simulink model "Simulation"  (R2023b)
settings: Solver=VariableStepAuto  StartTime=0.0  StopTime=1  RelTol=1e-3
values from neighbouring files (symbols this model uses):
  Adj = Adj1'    [graph_plot.m]
  G = digraph(Adj)    [graph_plot.m]
undefined symbols (not defined in the file or in its folder): A, B, c, C, F, K, Ko, L1, x0_0, xi_0
libraries: simulink x7
settings Model: Creator=fedpa  LastModifiedBy=fedpa

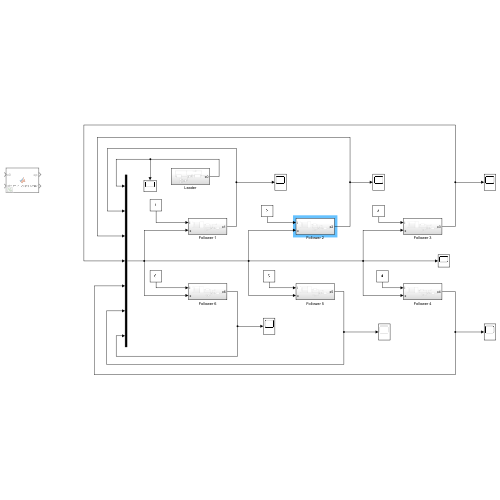
[thumbnail: Simulink's stored preview of the top-level diagram]
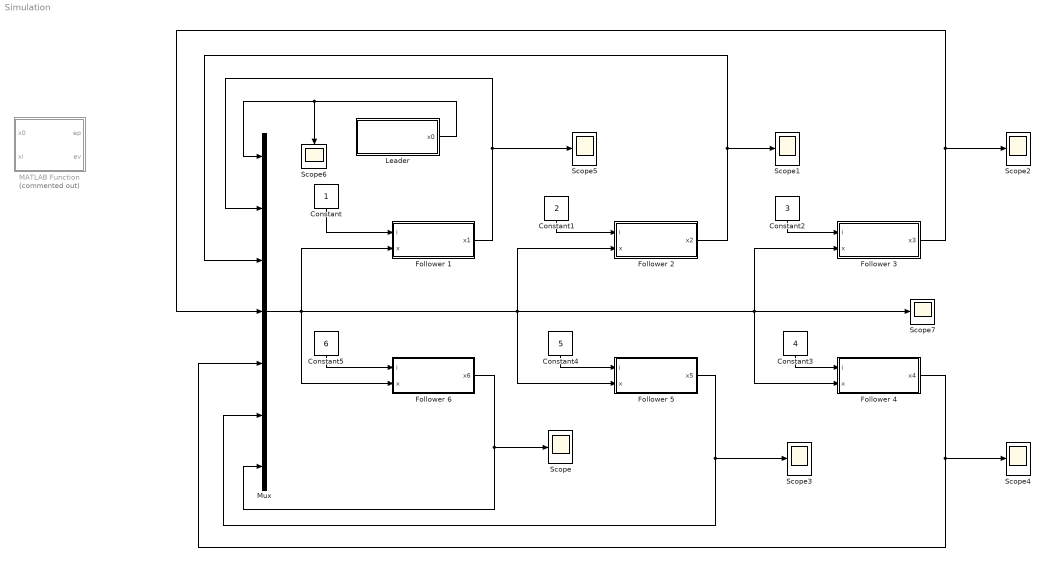
== system Simulation ==
  Constant : Constant
  Constant1 : Constant  Value=2
  Constant2 : Constant  Value=3
  Constant3 : Constant  Value=4
  Constant4 : Constant  Value=5
  Constant5 : Constant  Value=6
  Follower 1 : Subsystem
  Follower 2 : Subsystem
  Follower 3 : Subsystem
  Follower 4 : Subsystem
  Follower 5 : Subsystem
  Follower 6 : Subsystem
  Leader : Subsystem
  MATLAB Function : MATLAB Function  Commented=on  TreatAsAtomicUnit=on
  Mux : Mux  Inputs=7
  Scope{,1..7} (8 alike) : Scope
  wires:
  Constant3/1 -> Follower 4/1(i)
  Follower 3/1(x3) -> Scope2/1, Mux/4
  Follower 4/1(x4) -> Mux/5, Scope4/1
  Constant4/1 -> Follower 5/1(i)
  Constant5/1 -> Follower 6/1(i)
  Mux/1 -> Follower 1/2(x), Follower 5/2(x), Follower 2/2(x), Follower 4/2(x), Follower 3/2(x), Scope7/1, Follower 6/2(x)
  Follower 5/1(x5) -> Scope3/1, Mux/6
  Constant2/1 -> Follower 3/1(i)
  Follower 1/1(x1) -> Mux/2, Scope5/1
  Follower 2/1(x2) -> Mux/3, Scope1/1
  Constant/1 -> Follower 1/1(i)
  Constant1/1 -> Follower 2/1(i)
  Leader/1(x0) -> Mux/1, Scope6/1
  Follower 6/1(x6) -> Mux/7, Scope/1

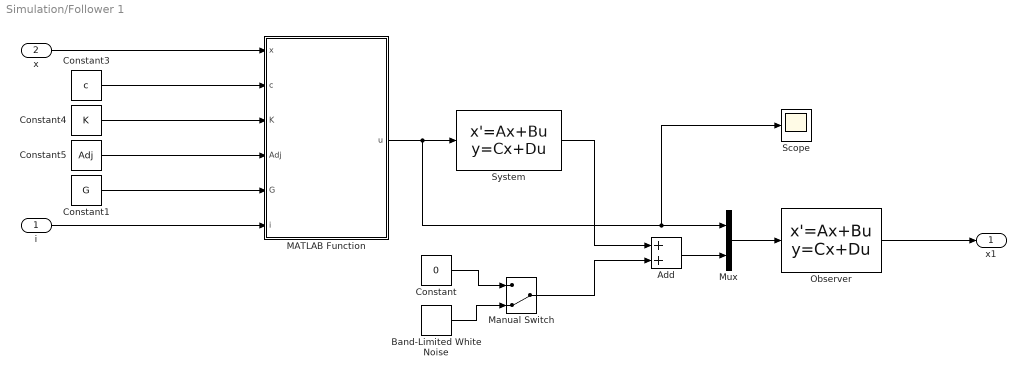
== system Simulation/Follower 1 ==
  i : Inport
  x : Inport  Port=2
  Add : Sum
  Band-Limited White Noise : simulink/Sources/Band-Limited White Noise  Cov=dis  Ts=0.1  seed=[23341]
  Constant : Constant  Value=0
  Constant1 : Constant  Value=G  VectorParams1D=off
  Constant3 : Constant  Value=c
  Constant4 : Constant  Value=K  VectorParams1D=off
  Constant5 : Constant  Value=Adj  VectorParams1D=off
  MATLAB Function : MATLAB Function  TreatAsAtomicUnit=on
  Manual Switch : ManualSwitch  CurrentSetting=0
  Mux : Mux  Inputs=2
  Observer : StateSpace  A=A-B*Ko-c*F*C  B=[B c*F]  C=eye(2)  D=zeros(2,2)  InitialCondition=0
  Scope : Scope
  System : StateSpace  A=A-B*Ko  B=B  C=C  D=0  InitialCondition=xi_0
  x1 : Outport
  wires:
  MATLAB Function/1(u) -> System/1, Scope/1, Mux/1
  Mux/1 -> Observer/1
  Observer/1 -> x1/1
  Constant4/1 -> MATLAB Function/3(K)
  i/1 -> MATLAB Function/6(i)
  Constant3/1 -> MATLAB Function/2(c)
  Constant1/1 -> MATLAB Function/5(G)
  Constant5/1 -> MATLAB Function/4(Adj)
  x/1 -> MATLAB Function/1(x)
  Add/1 -> Mux/2
  System/1 -> Add/1
  Manual Switch/1 -> Add/2
  Constant/1 -> Manual Switch/1
  Band-Limited White Noise/1 -> Manual Switch/2

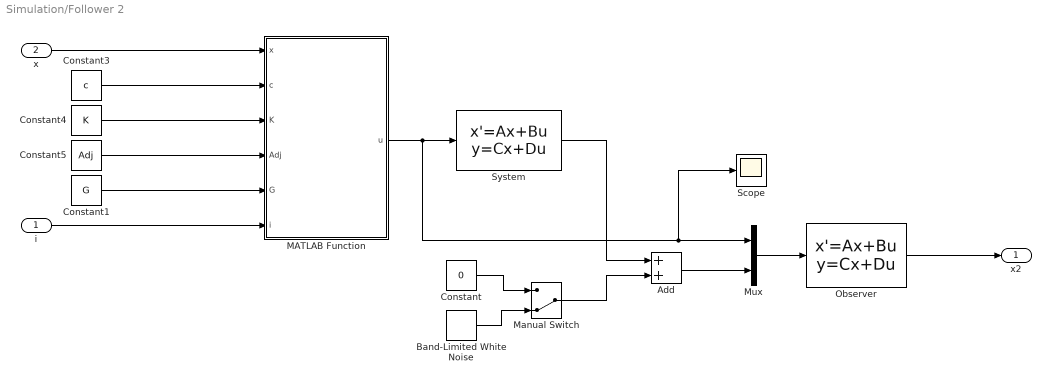
== system Simulation/Follower 2 ==
  i : Inport
  x : Inport  Port=2
  Add : Sum
  Band-Limited White Noise : simulink/Sources/Band-Limited White Noise  Cov=dis  Ts=0.1  seed=[23341]
  Constant : Constant  Value=0
  Constant1 : Constant  Value=G  VectorParams1D=off
  Constant3 : Constant  Value=c
  Constant4 : Constant  Value=K  VectorParams1D=off
  Constant5 : Constant  Value=Adj  VectorParams1D=off
  MATLAB Function : MATLAB Function  TreatAsAtomicUnit=on
  Manual Switch : ManualSwitch  CurrentSetting=0
  Mux : Mux  Inputs=2
  Observer : StateSpace  A=A-B*Ko-c*F*C  B=[B c*F]  C=eye(2)  D=zeros(2,2)  InitialCondition=0
  Scope : Scope
  System : StateSpace  A=A-B*Ko  B=B  C=C  D=0  InitialCondition=xi_0
  x2 : Outport
  wires:
  MATLAB Function/1(u) -> Scope/1, Mux/1, System/1
  Mux/1 -> Observer/1
  Observer/1 -> x2/1
  Constant4/1 -> MATLAB Function/3(K)
  i/1 -> MATLAB Function/6(i)
  Constant3/1 -> MATLAB Function/2(c)
  Constant1/1 -> MATLAB Function/5(G)
  Constant5/1 -> MATLAB Function/4(Adj)
  x/1 -> MATLAB Function/1(x)
  Add/1 -> Mux/2
  System/1 -> Add/1
  Manual Switch/1 -> Add/2
  Constant/1 -> Manual Switch/1
  Band-Limited White Noise/1 -> Manual Switch/2

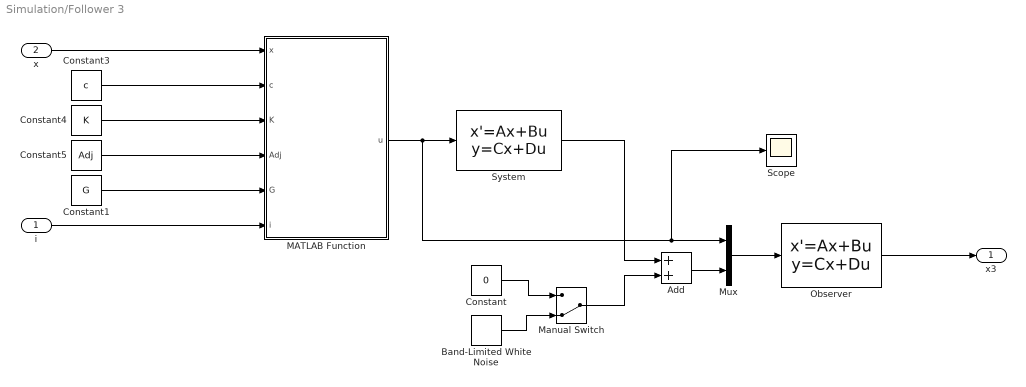
== system Simulation/Follower 3 ==
  i : Inport
  x : Inport  Port=2
  Add : Sum
  Band-Limited White Noise : simulink/Sources/Band-Limited White Noise  Cov=dis  Ts=0.1  seed=[23341]
  Constant : Constant  Value=0
  Constant1 : Constant  Value=G  VectorParams1D=off
  Constant3 : Constant  Value=c
  Constant4 : Constant  Value=K  VectorParams1D=off
  Constant5 : Constant  Value=Adj  VectorParams1D=off
  MATLAB Function : MATLAB Function  TreatAsAtomicUnit=on
  Manual Switch : ManualSwitch  CurrentSetting=0
  Mux : Mux  Inputs=2
  Observer : StateSpace  A=A-B*Ko-c*F*C  B=[B c*F]  C=eye(2)  D=zeros(2,2)  InitialCondition=0
  Scope : Scope
  System : StateSpace  A=A-B*Ko  B=B  C=C  D=0  InitialCondition=xi_0
  x3 : Outport
  wires:
  MATLAB Function/1(u) -> System/1, Scope/1, Mux/1
  Mux/1 -> Observer/1
  Observer/1 -> x3/1
  Constant4/1 -> MATLAB Function/3(K)
  i/1 -> MATLAB Function/6(i)
  Constant3/1 -> MATLAB Function/2(c)
  Constant1/1 -> MATLAB Function/5(G)
  Constant5/1 -> MATLAB Function/4(Adj)
  x/1 -> MATLAB Function/1(x)
  Add/1 -> Mux/2
  Manual Switch/1 -> Add/2
  System/1 -> Add/1
  Constant/1 -> Manual Switch/1
  Band-Limited White Noise/1 -> Manual Switch/2

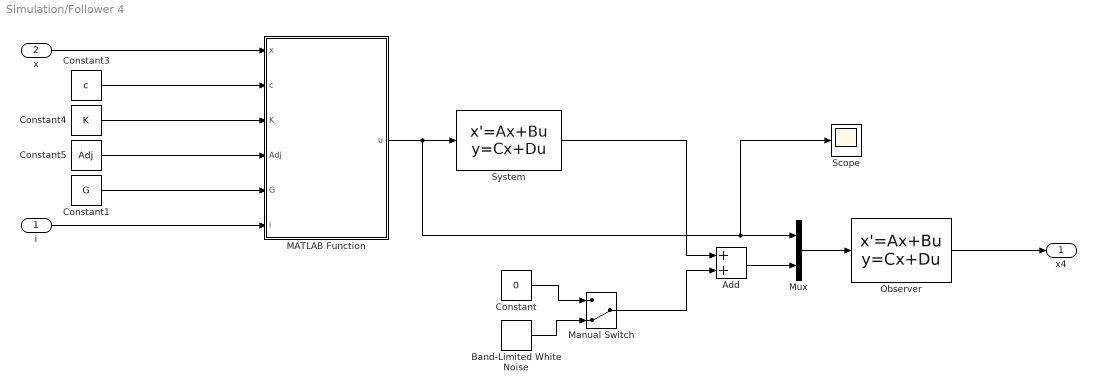
== system Simulation/Follower 4 ==
  i : Inport
  x : Inport  Port=2
  Add : Sum
  Band-Limited White Noise : simulink/Sources/Band-Limited White Noise  Cov=dis  Ts=0.1  seed=[23341]
  Constant : Constant  Value=0
  Constant1 : Constant  Value=G  VectorParams1D=off
  Constant3 : Constant  Value=c
  Constant4 : Constant  Value=K  VectorParams1D=off
  Constant5 : Constant  Value=Adj  VectorParams1D=off
  MATLAB Function : MATLAB Function  TreatAsAtomicUnit=on
  Manual Switch : ManualSwitch  CurrentSetting=0
  Mux : Mux  Inputs=2
  Observer : StateSpace  A=A-B*Ko-c*F*C  B=[B c*F]  C=eye(2)  D=zeros(2,2)  InitialCondition=0
  Scope : Scope
  System : StateSpace  A=A-B*Ko  B=B  C=C  D=0  InitialCondition=xi_0
  x4 : Outport
  wires:
  MATLAB Function/1(u) -> System/1, Scope/1, Mux/1
  Mux/1 -> Observer/1
  Observer/1 -> x4/1
  Constant4/1 -> MATLAB Function/3(K)
  i/1 -> MATLAB Function/6(i)
  Constant3/1 -> MATLAB Function/2(c)
  Constant1/1 -> MATLAB Function/5(G)
  Constant5/1 -> MATLAB Function/4(Adj)
  x/1 -> MATLAB Function/1(x)
  Manual Switch/1 -> Add/2
  Add/1 -> Mux/2
  System/1 -> Add/1
  Constant/1 -> Manual Switch/1
  Band-Limited White Noise/1 -> Manual Switch/2

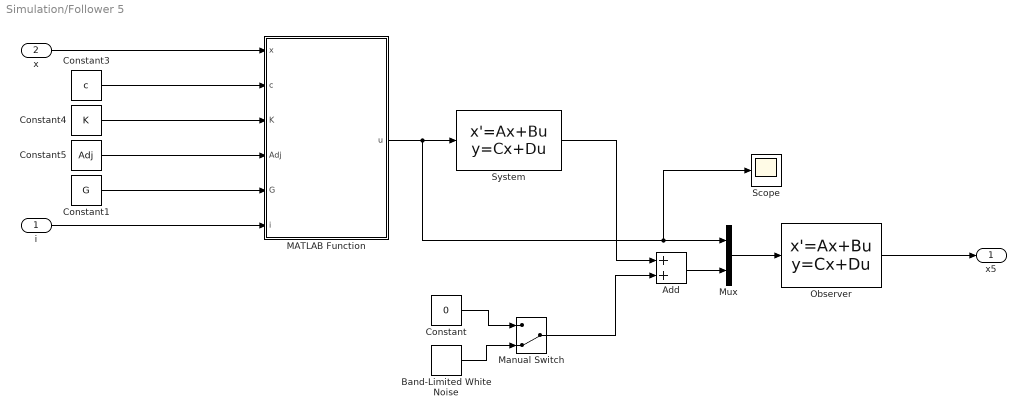
== system Simulation/Follower 5 ==
  i : Inport
  x : Inport  Port=2
  Add : Sum
  Band-Limited White Noise : simulink/Sources/Band-Limited White Noise  Cov=dis  Ts=0.1  seed=[23341]
  Constant : Constant  Value=0
  Constant1 : Constant  Value=G  VectorParams1D=off
  Constant3 : Constant  Value=c
  Constant4 : Constant  Value=K  VectorParams1D=off
  Constant5 : Constant  Value=Adj  VectorParams1D=off
  MATLAB Function : MATLAB Function  TreatAsAtomicUnit=on
  Manual Switch : ManualSwitch  CurrentSetting=0
  Mux : Mux  Inputs=2
  Observer : StateSpace  A=A-B*Ko-c*F*C  B=[B c*F]  C=eye(2)  D=zeros(2,2)  InitialCondition=0
  Scope : Scope
  System : StateSpace  A=A-B*Ko  B=B  C=C  D=0  InitialCondition=xi_0
  x5 : Outport
  wires:
  MATLAB Function/1(u) -> System/1, Scope/1, Mux/1
  Mux/1 -> Observer/1
  Observer/1 -> x5/1
  Constant4/1 -> MATLAB Function/3(K)
  i/1 -> MATLAB Function/6(i)
  Constant3/1 -> MATLAB Function/2(c)
  Constant1/1 -> MATLAB Function/5(G)
  Constant5/1 -> MATLAB Function/4(Adj)
  x/1 -> MATLAB Function/1(x)
  Add/1 -> Mux/2
  System/1 -> Add/1
  Constant/1 -> Manual Switch/1
  Band-Limited White Noise/1 -> Manual Switch/2
  Manual Switch/1 -> Add/2

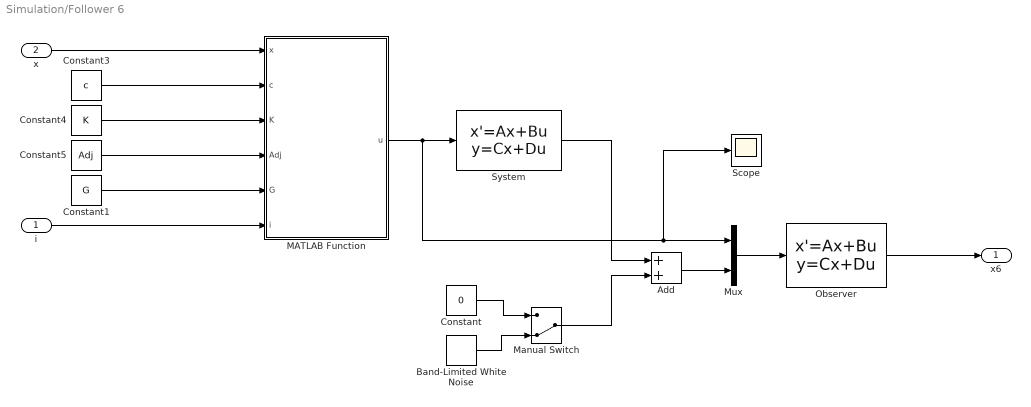
== system Simulation/Follower 6 ==
  i : Inport
  x : Inport  Port=2
  Add : Sum
  Band-Limited White Noise : simulink/Sources/Band-Limited White Noise  Cov=dis  Ts=0.1  seed=[23341]
  Constant : Constant  Value=0
  Constant1 : Constant  Value=G  VectorParams1D=off
  Constant3 : Constant  Value=c
  Constant4 : Constant  Value=K  VectorParams1D=off
  Constant5 : Constant  Value=Adj  VectorParams1D=off
  MATLAB Function : MATLAB Function  TreatAsAtomicUnit=on
  Manual Switch : ManualSwitch  CurrentSetting=0
  Mux : Mux  Inputs=2
  Observer : StateSpace  A=A-B*Ko-c*F*C  B=[B c*F]  C=eye(2)  D=zeros(2,2)  InitialCondition=0
  Scope : Scope
  System : StateSpace  A=A-B*Ko  B=B  C=C  D=0  InitialCondition=xi_0
  x6 : Outport
  wires:
  MATLAB Function/1(u) -> System/1, Scope/1, Mux/1
  Mux/1 -> Observer/1
  Observer/1 -> x6/1
  Constant4/1 -> MATLAB Function/3(K)
  i/1 -> MATLAB Function/6(i)
  Constant3/1 -> MATLAB Function/2(c)
  Constant1/1 -> MATLAB Function/5(G)
  Constant5/1 -> MATLAB Function/4(Adj)
  x/1 -> MATLAB Function/1(x)
  Manual Switch/1 -> Add/2
  Add/1 -> Mux/2
  System/1 -> Add/1
  Constant/1 -> Manual Switch/1
  Band-Limited White Noise/1 -> Manual Switch/2

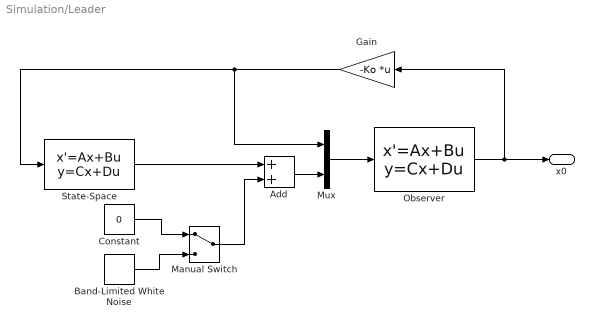
== system Simulation/Leader ==
  Add : Sum
  Band-Limited White Noise : simulink/Sources/Band-Limited White Noise  Cov=dis  Ts=0.1  seed=[23341]
  Constant : Constant  Value=0
  Gain : Gain  Gain=-Ko  Multiplication=Matrix(K*u)
  Manual Switch : ManualSwitch
  Mux : Mux  Inputs=2
  Observer : StateSpace  A=A-L1*C  B=[B L1]  C=eye(2)  D=zeros(2,2)  InitialCondition=0
  State-Space : StateSpace  A=A  B=B  C=C  D=0  InitialCondition=x0_0
  x0 : Outport
  wires:
  Gain/1 -> State-Space/1, Mux/1
  Observer/1 -> Gain/1, x0/1
  Mux/1 -> Observer/1
  State-Space/1 -> Add/1
  Add/1 -> Mux/2
  Manual Switch/1 -> Add/2
  Band-Limited White Noise/1 -> Manual Switch/2
  Constant/1 -> Manual Switch/1

== matlab function Simulation/Follower 2/MATLAB Function ==
  data: x input; u output; c input; K input; Adj input; G input; i input
function u = controller(x, c, K, Adj, G, i)
    epsi = zeros(2,1);
    sub = G(i,i)*(x(1:2)-x(i*2+1:i*2+2));
    for j = 1:6
        epsi = epsi + Adj(i,j)*(x(j*2+1:j*2+2)-x(i*2+1:i*2+2));
    end
    epsi = epsi+sub;
    
    u = c*K*epsi;
end

== matlab function Simulation/Follower 1/MATLAB Function ==
  data: x input; u output; c input; K input; Adj input; G input; i input
function u = controller(x, c, K, Adj, G, i)
    epsi = zeros(2,1);
    sub = G(i,i)*(x(1:2)-x(i*2+1:i*2+2));
    for j = 1:6
        epsi = epsi + Adj(i,j)*(x(j*2+1:j*2+2)-x(i*2+1:i*2+2));
    end
    epsi = epsi+sub;
    
    u = c*K*epsi;
end

== matlab function Simulation/Follower 3/MATLAB Function ==
  data: x input; u output; c input; K input; Adj input; G input; i input
function u = controller(x, c, K, Adj, G, i)
    epsi = zeros(2,1);
    sub = G(i,i)*(x(1:2)-x(i*2+1:i*2+2));
    for j = 1:6
        epsi = epsi + Adj(i,j)*(x(j*2+1:j*2+2)-x(i*2+1:i*2+2));
    end
    epsi = epsi+sub;
    
    u = c*K*epsi;
end

== matlab function Simulation/Follower 4/MATLAB Function ==
  data: x input; u output; c input; K input; Adj input; G input; i input
function u = controller(x, c, K, Adj, G, i)
    epsi = zeros(2,1);
    sub = G(i,i)*(x(1:2)-x(i*2+1:i*2+2));
    for j = 1:6
        epsi = epsi + Adj(i,j)*(x(j*2+1:j*2+2)-x(i*2+1:i*2+2));
    end
    epsi = epsi+sub;
    
    u = c*K*epsi;
end

== matlab function Simulation/Follower 5/MATLAB Function ==
  data: x input; u output; c input; K input; Adj input; G input; i input
function u = controller(x, c, K, Adj, G, i)
    epsi = zeros(2,1);
    sub = G(i,i)*(x(1:2)-x(i*2+1:i*2+2));
    for j = 1:6
        epsi = epsi + Adj(i,j)*(x(j*2+1:j*2+2)-x(i*2+1:i*2+2));
    end
    epsi = epsi+sub;
    
    u = c*K*epsi;
end

== matlab function Simulation/Follower 6/MATLAB Function ==
  data: x input; u output; c input; K input; Adj input; G input; i input
function u = controller(x, c, K, Adj, G, i)
    epsi = zeros(2,1);
    sub = G(i,i)*(x(1:2)-x(i*2+1:i*2+2));
    for j = 1:6
        epsi = epsi + Adj(i,j)*(x(j*2+1:j*2+2)-x(i*2+1:i*2+2));
    end
    epsi = epsi+sub;
    
    u = c*K*epsi;
end

== matlab function Simulation/MATLAB Function ==
  data: x0 input; ep output; xi input; ev output
function [ep, ev] = norm2_distance(x0, xi)
    ep = norm(x0(1)-xi(1));
    ev = norm(x0(2)-xi(2));
end
